simulink model "Plant2"  (R2015b)
settings: Solver=ode45  StartTime=0.0  StopTime=10.0  MaxStep=0.01  RelTol=1e-5
values from neighbouring files (symbols this model uses):
  GDyskretne = acker(systemDyskretny.A',systemDyskretny.C',[exp(T*-14),exp(T*-28),exp(T*-36)])'    [zad1.m]
  systemDyskretny = c2d(system,T,'foh')    [zad1.m]
settings Model: Creator=Szwank  LastModifiedBy=student
settings DataIOCC: SaveFormat=Array
settings DebuggingCC: SolverPrmCheckMsg=warning
settings HardwareCC: ProdBitPerPointer=32  ProdLargestAtomicFloat=None  ProdIntDivRoundTo=Undefined  ProdEndianess=Unspecified  ProdWordSize=32  ProdHWDeviceType=32-bit Generic
settings GRTTargetCC: GeneratePreprocessorConditionals=Disable all
settings ConfigComp: CovModelRefEnable=Off  CovSFcnEnable=off

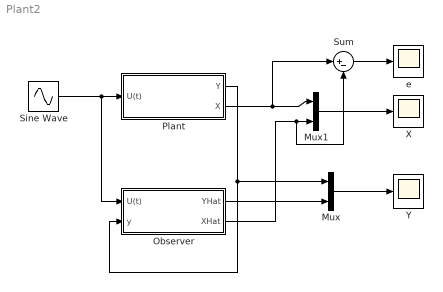
== system Plant2 ==
  Mux : Mux  Inputs=2
  Mux1 : Mux  Inputs=2
  "Observer " : Subsystem
  Plant : Subsystem
  Sine Wave : Sin  SampleTime=0
  Sum : Sum  Inputs=|+-
  X : Scope
  Y : Scope
  e : Scope
  wires:
  Sine Wave/1 -> "Observer "/1(U(t)), Plant/1(U(t))
  Plant/1(Y) -> Mux/1, "Observer "/2("y ")
  "Observer "/1(YHat) -> Mux/2
  Plant/2(X) -> Sum/1, Mux1/1
  "Observer "/2(XHat) -> Sum/2, Mux1/2
  Mux1/1 -> X/1
  Mux/1 -> Y/1
  Sum/1 -> e/1

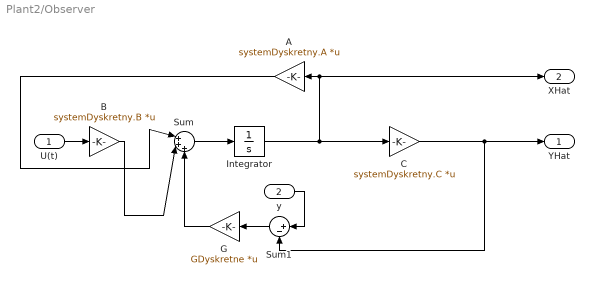
== system Plant2/Observer  ==
  U(t) : Inport
  "y " : Inport  Port=2
  A : Gain  Gain=systemDyskretny.A  Multiplication=Matrix(K*u)
  B : Gain  Gain=systemDyskretny.B  Multiplication=Matrix(K*u)
  C : Gain  Gain=systemDyskretny.C  Multiplication=Matrix(K*u)
  G : Gain  Gain=GDyskretne  Multiplication=Matrix(K*u)
  Integrator : Integrator
  Sum : Sum  Inputs=|+++
  Sum1 : Sum  Inputs=|+-
  YHat : Outport
  XHat : Outport  Port=2
  wires:
  A/1 -> Sum/1
  U(t)/1 -> B/1
  Integrator/1 -> C/1, XHat/1, A/1
  C/1 -> Sum1/2, YHat/1
  B/1 -> Sum/2
  Sum/1 -> Integrator/1
  "y "/1 -> Sum1/1
  Sum1/1 -> G/1
  G/1 -> Sum/3

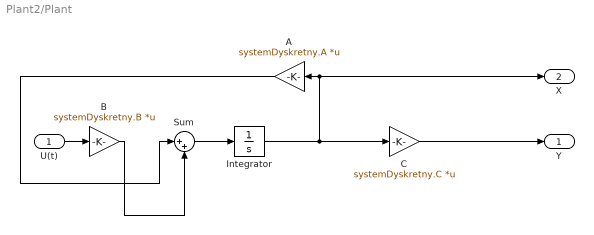
== system Plant2/Plant ==
  U(t) : Inport
  A : Gain  Gain=systemDyskretny.A  Multiplication=Matrix(K*u)
  B : Gain  Gain=systemDyskretny.B  Multiplication=Matrix(K*u)
  C : Gain  Gain=systemDyskretny.C  Multiplication=Matrix(K*u)
  Integrator : Integrator
  Sum : Sum  Inputs=|++
  Y : Outport
  X : Outport  Port=2
  wires:
  A/1 -> Sum/1
  U(t)/1 -> B/1
  Integrator/1 -> C/1, X/1, A/1
  C/1 -> Y/1
  B/1 -> Sum/2
  Sum/1 -> Integrator/1
